simulink model "InnerTrans"  (R2020b)
settings: Solver=VariableStepAuto  StartTime=0.0  StopTime=10.0  RelTol=1e-3
settings Model: EnablePacing=on  PacingRate=0.500000  Creator=apple  LastModifiedBy=apple

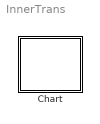
== system InnerTrans ==
  Chart : Stateflow chart  TreatAsAtomicUnit=on

== stateflow chart InnerTrans/Chart ==
  state A
    en:fprintf("enA");
    du:x = x+1;
    ex:fprintf("exA");
    state A1
    state A2
    (default) -> A1
    A2 -> A1 : {x = x-1;}
    A1 -> A2 : {x = x+1;}
    A -> A [order 1] : [x>1]{x = x+1;}
  (default) -> A : {x = 0;}
  A -> A [order 1] : [x>3]{x=0;}
  data: x local
